simulink model "WTPG"  (R2022a)
settings: Solver=FixedStepDiscrete  StartTime=0.0  StopTime=10  FixedStep=0.04  RelTol=1e-3  EnableMultiTasking=on
PreLoadFcn:
  | listing = dir;
  | if (contains([listing .name], 'TCAF')) && (contains([listing .name], 'MAP'))
  |     addpath('./TCAF', './MAP');
  |     addpath( genpath('./MAP') );
  | elseif (contains([listing .name], 'WTPG.slx'))
  |     addpath('../TCAF', '../MAP');
  |     addpath( genpath('../MAP') );
  | else
  | 
  | end
  | 
  | load('BusStructureWTPG.mat');
  | load('TRN\BusStructureTRN.mat');
InitFcn:
  | listing = dir;
  | if (contains([listing .name], 'TCAF')) && (contains([listing .name], 'MAP'))
  |     addpath('./TCAF', './MAP');
  |     addpath( genpath('./MAP') );
  | elseif (contains([listing .name], 'WTPG.slx'))
  |     addpath('../TCAF', '../MAP');
  |     addpath( genpath('../MAP') );
  | else
  | 
  | end
  | 
  | load('BusStructureWTPG.mat');
  | load('TRN\BusStructureTRN.mat');
values from neighbouring files (symbols this model uses):
  isFeasible = logsout{idx_WTPGDatapump}.Values.isFeasible.Data(ii,:)    [WTPG_SIM_AFTERPLOT.m]
  wtpgOffTerMap = logsout{idx_WTPGOutput}.Values.wtpgOffTerMap.Data(ii,:)    [WTPG_SIM_AFTERPLOT.m]
  wtpgValid = logsout{idx_WTPGOutput}.Values.wtpgValid.Data(ii)    [WTPG_SIM_AFTERPLOT.m]
undefined symbols (not defined in the file or in its folder): predictedTrajectory, wtp, wtpgOffObsMap, wtpValid
libraries: simulink x1
settings Model: Creator=ASCL  LastModifiedBy=ASCL
settings SolverCC: AutoInsertRateTranBlk=on
settings DataIOCC: SaveOutput=off  SignalLogging=off  DSMLogging=off  SaveTime=off  ReturnWorkspaceOutputs=off
settings OptimizationCC: BlockReduction=off  DefaultParameterBehavior=Inlined  UseDivisionForNetSlopeComputation=on  GainParamInheritBuiltInType=on  UseFloatMulNetSlope=on  ExpressionFolding=off  PassReuseOutputArgsAs=Individual arguments  ZeroExternalMemoryAtStartup=off  ZeroInternalMemoryAtStartup=off  EfficientFloat2IntCast=on  LifeSpan=inf  OptimizeBlockOrder=speed  DifferentSizesBufferReuse=on  EfficientTunableParamExpr=on
settings DebuggingCC: SignalInfNanChecking=warning  ReadBeforeWriteMsg=EnableAllAsError  WriteAfterWriteMsg=EnableAllAsError  WriteAfterReadMsg=EnableAllAsError  IntegerOverflowMsg=error  ParameterTunabilityLossMsg=error  UniqueDataStoreMsg=error  AssertControl=DisableAll  NonBusSignalsTreatedAsBus=error  SFInvalidInputDataAccessInChartInitDiag=error  SFTransitionOutsideNaturalParentDiag=error  SFUnreachableExecutionPathDiag=error  SFUndirectedBroadcastEventsDiag=error  IntegerSaturationMsg=error
settings HardwareCC: ProdBitPerPointer=32  ProdBitPerSizeT=32  ProdBitPerPtrDiffT=32  ProdLargestAtomicInteger=Long  ProdLargestAtomicFloat=Double  ProdEndianess=BigEndian  ProdWordSize=32  ProdLongLongMode=on  ProdHWDeviceType=Freescale->MPC83xx
settings ModelReferenceCC: ModelReferenceNumInstancesAllowed=Single
settings SFSimCC: SimCustomHeaderCode="#include \"MAP.h\""  SimUserSources=MAP.c  SimUserLibraries=WS2_32.LIB  CompileTimeRecursionLimit=0  EnableRuntimeRecursion=off  MATLABDynamicMemAlloc=off
settings RTWCC: SystemTargetFile=ert.tlc  TemplateMakefile=ert_default_tmf  GenerateReport=on  RTWUseSimCustomCode=on  CustomHeaderCode="#include \"MAP.h\""  CustomSource=MAP.c  CustomLibrary=WS2_32.LIB  BuildConfiguration=Faster Runs  IncludeHyperlinkInReport=on  LaunchReport=on  GenerateTraceInfo=on  GenerateTraceReport=on  GenerateTraceReportSl=on  GenerateTraceReportSf=on  GenerateTraceReportEml=on  GenerateCodeMetricsReport=on
settings CodeAppCC: ForceParamTrailComments=on  IgnoreCustomStorageClasses=off  OperatorAnnotations=on  SimulinkDataObjDesc=on  SFDataObjDesc=on  MATLABFcnDesc=on  InsertBlockDesc=on  StateflowObjectComments=on  MATLABSourceComments=on  EnableCustomComments=on  InlinedPrmAccess=Macros  ReqsInCode=on
settings ERTTargetCC: TargetLangStandard=C99 (ISO)  UtilityFuncGeneration=Shared location  GenerateSampleERTMain=on  IncludeMdlTerminateFcn=off  CombineSignalStateStructs=on  SuppressErrorStatus=on  SupportAbsoluteTime=off  SupportNonFinite=off  SupportComplex=off  SupportVariableSizeSignals=on  ParenthesesLevel=Standards  CastingMode=Standards  GenerateSharedConstants=off  InlinedParameterPlacement=NonHierarchical  ERTCustomFileTemplate=example_file_process.tlc  RateTransitionBlockCode=Function  PreserveIfCondition=on  ConvertIfToSwitch=off  EnableSignedLeftShifts=off  EnableSignedRightShifts=off

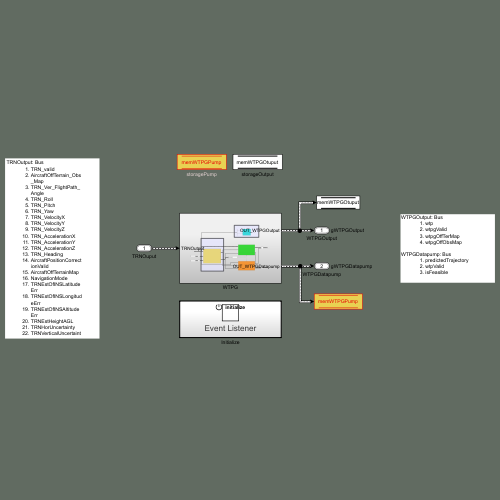
[thumbnail: Simulink's stored preview of the top-level diagram]
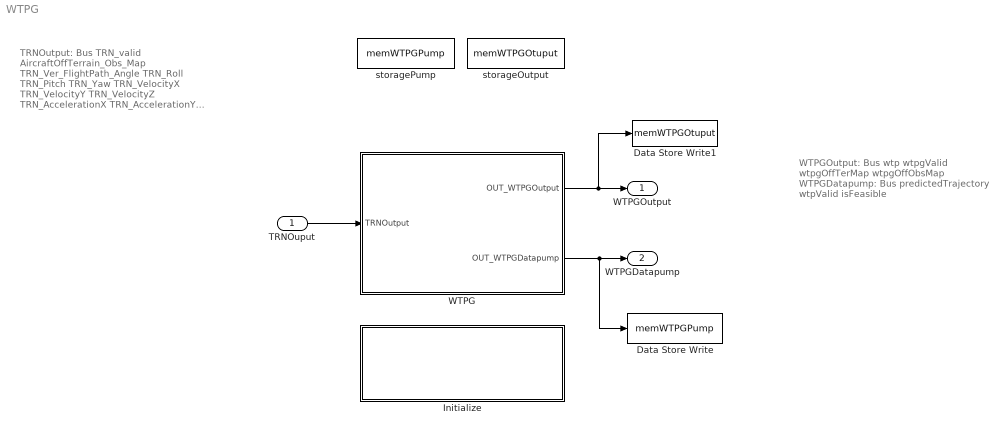
== system WTPG ==
  note: TRNOutput: Bus
      | TRN_valid
      | AircraftOffTerrain_Obs_Map
      | TRN_Ver_FlightPath_Angle
      | TRN_Roll
      | TRN_Pitch
      | TRN_Yaw
      | TRN_VelocityX
      | TRN_VelocityY
      | TRN_VelocityZ
      | TRN_AccelerationX
      | TRN_AccelerationY
      | TRN_AccelerationZ
      | TRN_Heading
      | AircraftPositionCorrectionValid
      | AircraftOffTerrainMap
      | NavigationMode
      | TRNEstOfINSLatitudeErr
      | TRNEstOfINSLongitudeErr
      | TRNEstOfINSAltitudeErr
      | TRNEstHeightAGL
      | TRNHorUncertainty
      | TRNVerticalUncertainty
      | TRNTimeTag
      | Latitude_INS
      | Longitude_INS
      | Altitude_INS
  note: WTPGOutput: Bus
      | wtp
      | wtpgValid
      | wtpgOffTerMap
      | wtpgOffObsMap
      |
      | WTPGDatapump: Bus
      | predictedTrajectory
      | wtpValid
      | isFeasible
  TRNOuput : Inport  OutDataTypeStr=Bus: TRNOutput  SampleTime=0.04  Interpolate=off  BusOutputAsStruct=on
  Data Store Write : DataStoreWrite  DataStoreName=memWTPGPump  IndexOptions=Index vector (dialog)  Indices=1  OutputSizes=1
  Data Store Write1 : DataStoreWrite  DataStoreName=memWTPGOtuput  IndexOptions=Index vector (dialog)  Indices=1  OutputSizes=1
  Initialize : Subsystem  TreatAsAtomicUnit=on
  WTPG : Subsystem
  storageOutput : DataStoreMemory  DataStoreName=memWTPGOtuput  WriteAfterWriteMsg=warning  VectorParams1D=off  ShowAdditionalParam=off  OutDataTypeStr=Bus: WTPGOutput
      settings: LockScale=on
  storagePump : DataStoreMemory  DataStoreName=memWTPGPump  WriteAfterWriteMsg=warning  VectorParams1D=off  ShowAdditionalParam=off  OutDataTypeStr=Bus: WTPGDatapump
      settings: LockScale=on
  WTPGOutput : Outport  SignalName=gWTPGOutput  OutDataTypeStr=Bus: WTPGOutput  SampleTime=0.04  BusOutputAsStruct=on
  WTPGDatapump : Outport  Port=2  SignalName=gWTPGDatapump  OutDataTypeStr=Bus: WTPGDatapump  SampleTime=0.04  BusOutputAsStruct=on
  wires:
  TRNOuput/1 -> WTPG/1(TRNOutput)
  WTPG/1(OUT_WTPGOutput) -> Data Store Write1/1, WTPGOutput/1
  WTPG/2(OUT_WTPGDatapump) -> Data Store Write/1, WTPGDatapump/1

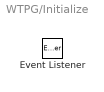
== system WTPG/Initialize ==
  Event Listener : EventListener  DisableCoverage=on  EventName=reset

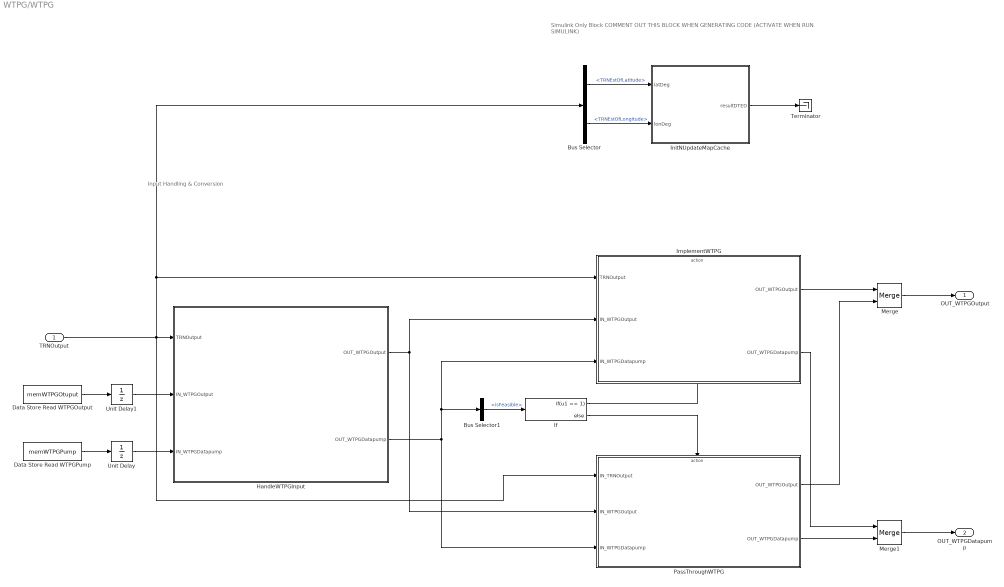
== system WTPG/WTPG ==
  note: Simulink Only Block
      | COMMENT OUT THIS BLOCK WHEN GENERATING CODE
      | (ACTIVATE WHEN RUN SIMULINK)
  note: Input Handling & Conversion
  TRNOutput : Inport  OutDataTypeStr=Bus: TRNOutput
  Bus Selector : BusSelector  OutputSignals=TRNEstOfLatitude,TRNEstOfLongitude
  Bus Selector1 : BusSelector  OutputSignals=isFeasible
  Data Store Read WTPGPump : DataStoreRead  DataStoreName=memWTPGPump  IndexOptions=Index vector (dialog)  Indices=1  OutputSizes=1
  Data Store Read WTPGOutput : DataStoreRead  DataStoreName=memWTPGOtuput  IndexOptions=Index vector (dialog)  Indices=1  OutputSizes=1
  HandleWTPGInput : Subsystem  TreatAsAtomicUnit=on
      settings: RTWSystemCode=Nonreusable function  RTWFcnNameOpts=Use subsystem name  FunctionInterfaceSpec=Allow arguments (Optimized)
  If : If  IfExpression=u1 == 1
  ImplementWTPG : Subsystem
      settings: RTWSystemCode=Nonreusable function  RTWFcnNameOpts=Use subsystem name
  InitNUpdateMapCache : Subsystem  TreatAsAtomicUnit=on
  Merge : Merge
  Merge1 : Merge
  PassThroughWTPG : Subsystem  TreatAsAtomicUnit=on
      settings: RTWSystemCode=Nonreusable function  RTWFcnNameOpts=Use subsystem name
  Terminator : Terminator
  Unit Delay : UnitDelay  SampleTime=-1  HasFrameUpgradeWarning=on
  Unit Delay1 : UnitDelay  SampleTime=-1  HasFrameUpgradeWarning=on
  OUT_WTPGOutput : Outport  OutDataTypeStr=Bus: WTPGOutput  SampleTime=0.04
  OUT_WTPGDatapump : Outport  Port=2  OutDataTypeStr=Bus: WTPGDatapump  SampleTime=0.04
  wires:
  InitNUpdateMapCache/1(resultDTED) -> Terminator/1
  ImplementWTPG/1(OUT_WTPGOutput) -> Merge/1
  ImplementWTPG/2(OUT_WTPGDatapump) -> Merge1/1
  Bus Selector/1 -> InitNUpdateMapCache/1(latDeg)  "<TRNEstOfLatitude>"
  Bus Selector/2 -> InitNUpdateMapCache/2(lonDeg)  "<TRNEstOfLongitude>"
  Data Store Read WTPGOutput/1 -> Unit Delay1/1
  Data Store Read WTPGPump/1 -> Unit Delay/1
  Unit Delay1/1 -> HandleWTPGInput/2(IN_WTPGOutput)
  Unit Delay/1 -> HandleWTPGInput/3(IN_WTPGDatapump)
  HandleWTPGInput/2(OUT_WTPGDatapump) -> ImplementWTPG/3(IN_WTPGDatapump), Bus Selector1/1, PassThroughWTPG/3(IN_WTPGDatapump)
  HandleWTPGInput/1(OUT_WTPGOutput) -> ImplementWTPG/2(IN_WTPGOutput), PassThroughWTPG/2(IN_WTPGOutput)
  Bus Selector1/1 -> If/1  "<isFeasible>"
  If/2 -> PassThroughWTPG/Action
  If/1 -> ImplementWTPG/Action
  TRNOutput/1 -> PassThroughWTPG/1(IN_TRNOutput), Bus Selector/1, ImplementWTPG/1(TRNOutput), HandleWTPGInput/1(TRNOutput)
  PassThroughWTPG/1(OUT_WTPGOutput) -> Merge/2
  Merge/1 -> OUT_WTPGOutput/1
  PassThroughWTPG/2(OUT_WTPGDatapump) -> Merge1/2
  Merge1/1 -> OUT_WTPGDatapump/1

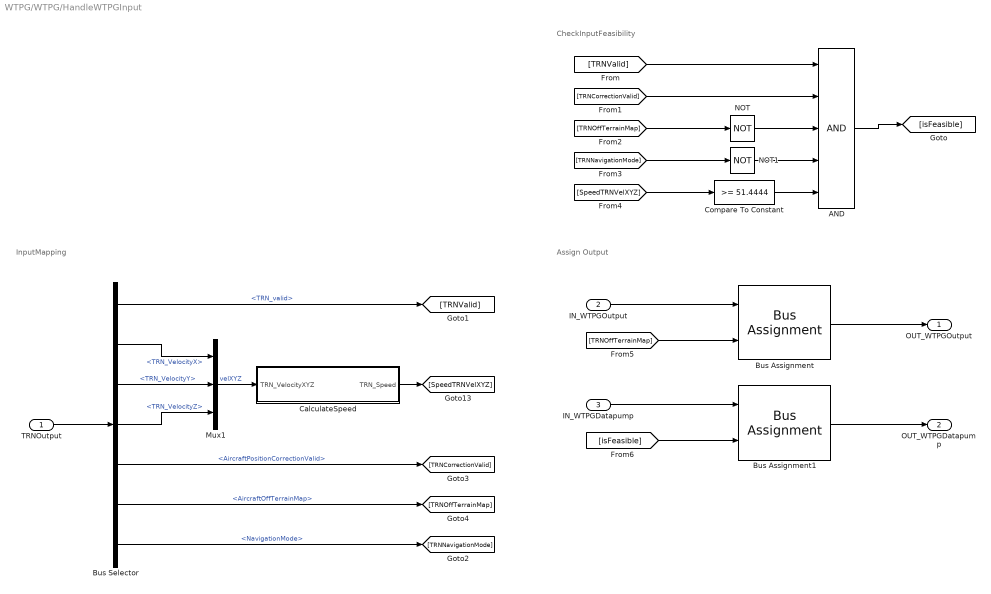
== system WTPG/WTPG/HandleWTPGInput ==
  note: Assign Output
  note: CheckInputFeasibility
  note: InputMapping
  TRNOutput : Inport  OutDataTypeStr=Bus: TRNOutput  SampleTime=0.04
  IN_WTPGOutput : Inport  Port=2
  IN_WTPGDatapump : Inport  Port=3
  AND : Logic  Inputs=5  AllPortsSameDT=off  OutDataTypeStr=boolean
  Bus Assignment : BusAssignment  AssignedSignals=wtpgOffTerMap
  Bus Assignment1 : BusAssignment  AssignedSignals=isFeasible
  Bus Selector : BusSelector  OutputSignals=TRN_valid,TRN_VelocityX,TRN_VelocityY,TRN_VelocityZ,AircraftPositionCorrectionValid,AircraftOffTerrainMap,NavigationMode
  CalculateSpeed : Subsystem
  Compare To Constant : simulink/Logic and Bit Operations/Compare To Constant  relop=>=  const=51.4444  OutDataTypeStr=boolean
  Mux1 : Mux  Inputs=3
  NOT : Logic  Operator=NOT  AllPortsSameDT=off  OutDataTypeStr=boolean
  NOT1 : Logic  Operator=NOT  AllPortsSameDT=off  OutDataTypeStr=boolean
  OUT_WTPGOutput : Outport
  OUT_WTPGDatapump : Outport  Port=2
  wires:
  TRNOutput/1 -> Bus Selector/1
  Bus Selector/2 -> Mux1/1  "<TRN_VelocityX>"
  Mux1/1 -> CalculateSpeed/1(TRN_VelocityXYZ)  "velXYZ"
  Bus Selector/4 -> Mux1/3  "<TRN_VelocityZ>"
  Bus Selector/3 -> Mux1/2  "<TRN_VelocityY>"
  Bus Selector/1 -> [TRNValid]  "<TRN_valid>"
  Bus Selector/5 -> [TRNCorrectionValid]  "<AircraftPositionCorrectionValid>"
  Bus Selector/6 -> [TRNOffTerrainMap]  "<AircraftOffTerrainMap>"
  Bus Selector/7 -> [TRNNavigationMode]  "<NavigationMode>"
  [TRNOffTerrainMap] -> NOT/1
  [TRNValid] -> AND/1
  [TRNCorrectionValid] -> AND/2
  NOT/1 -> AND/3
  [TRNNavigationMode] -> NOT1/1
  AND/1 -> [isFeasible]
  NOT1/1 -> AND/4
  CalculateSpeed/1(TRN_Speed) -> [SpeedTRNVelXYZ]
  [SpeedTRNVelXYZ] -> Compare To Constant/1
  Compare To Constant/1 -> AND/5
  IN_WTPGOutput/1 -> Bus Assignment/1
  Bus Assignment/1 -> OUT_WTPGOutput/1
  [TRNOffTerrainMap] -> Bus Assignment/2
  IN_WTPGDatapump/1 -> Bus Assignment1/1
  Bus Assignment1/1 -> OUT_WTPGDatapump/1
  [isFeasible] -> Bus Assignment1/2

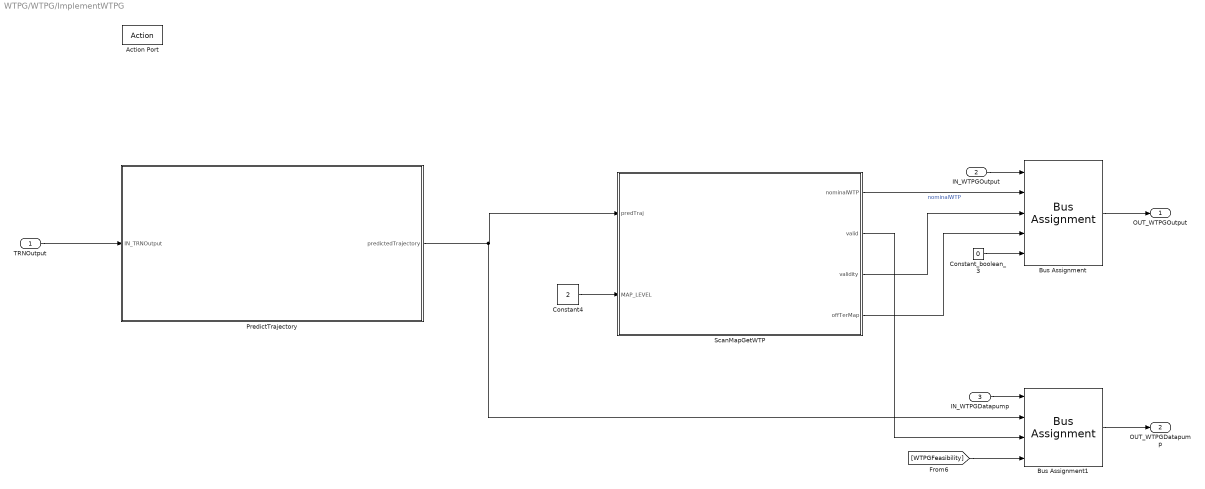
== system WTPG/WTPG/ImplementWTPG ==
  TRNOutput : Inport
  IN_WTPGOutput : Inport  Port=2  OutDataTypeStr=Bus: WTPGOutput
  IN_WTPGDatapump : Inport  Port=3  OutDataTypeStr=Bus: WTPGDatapump
  Action Port : ActionPort  ActionPortLabel=if(u1 == 1)
  Bus Assignment : BusAssignment  AssignedSignals=wtp,wtpgValid,wtpgOffTerMap,wtpgOffObsMap
  Bus Assignment1 : BusAssignment  AssignedSignals=predictedTrajectory,wtpValid,isFeasible
  Constant4 : Constant  Value=2  OutDataTypeStr=uint16  SampleTime=0.04
  Constant_boolean_3 : Constant  Value=0  OutDataTypeStr=boolean  SampleTime=0.04
  PredictTrajectory : Subsystem
  ScanMapGetWTP : MATLAB Function  TreatAsAtomicUnit=on  SystemSampleTime=0.04
      settings: RTWSystemCode=Nonreusable function  RTWFcnNameOpts=Use subsystem name
  OUT_WTPGOutput : Outport  OutDataTypeStr=Bus: WTPGOutput
  OUT_WTPGDatapump : Outport  Port=2  OutDataTypeStr=Bus: WTPGDatapump  SampleTime=0.04
  wires:
  ScanMapGetWTP/3(validity) -> Bus Assignment/3
  PredictTrajectory/1(predictedTrajectory) -> Bus Assignment1/2, ScanMapGetWTP/1(predTraj)
  Constant4/1 -> ScanMapGetWTP/2(MAP_LEVEL)
  Bus Assignment/1 -> OUT_WTPGOutput/1
  ScanMapGetWTP/1(nominalWTP) -> Bus Assignment/2  "nominalWTP"
  Constant_boolean_3/1 -> Bus Assignment/5
  ScanMapGetWTP/4(offTerMap) -> Bus Assignment/4
  IN_WTPGOutput/1 -> Bus Assignment/1
  IN_WTPGDatapump/1 -> Bus Assignment1/1
  [WTPGFeasibility] -> Bus Assignment1/4
  Bus Assignment1/1 -> OUT_WTPGDatapump/1
  ScanMapGetWTP/2(valid) -> Bus Assignment1/3
  TRNOutput/1 -> PredictTrajectory/1(IN_TRNOutput)

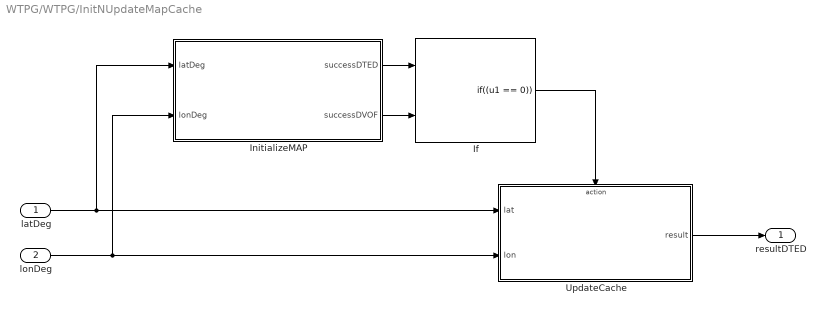
== system WTPG/WTPG/InitNUpdateMapCache ==
  latDeg : Inport  OutDataTypeStr=double
  lonDeg : Inport  Port=2  OutDataTypeStr=double
  If : If  NumInputs=2  IfExpression=(u1 == 0)  ShowElse=off
  InitializeMAP : MATLAB Function  TreatAsAtomicUnit=on
  UpdateCache : Subsystem  TreatAsAtomicUnit=on
  resultDTED : Outport  VectorParamsAs1DForOutWhenUnconnected=off
  wires:
  lonDeg/1 -> InitializeMAP/2(lonDeg), UpdateCache/2(lon)
  UpdateCache/1(result) -> resultDTED/1
  InitializeMAP/1(successDTED) -> If/1
  latDeg/1 -> InitializeMAP/1(latDeg), UpdateCache/1(lat)
  InitializeMAP/2(successDVOF) -> If/2
  If/1 -> UpdateCache/Action

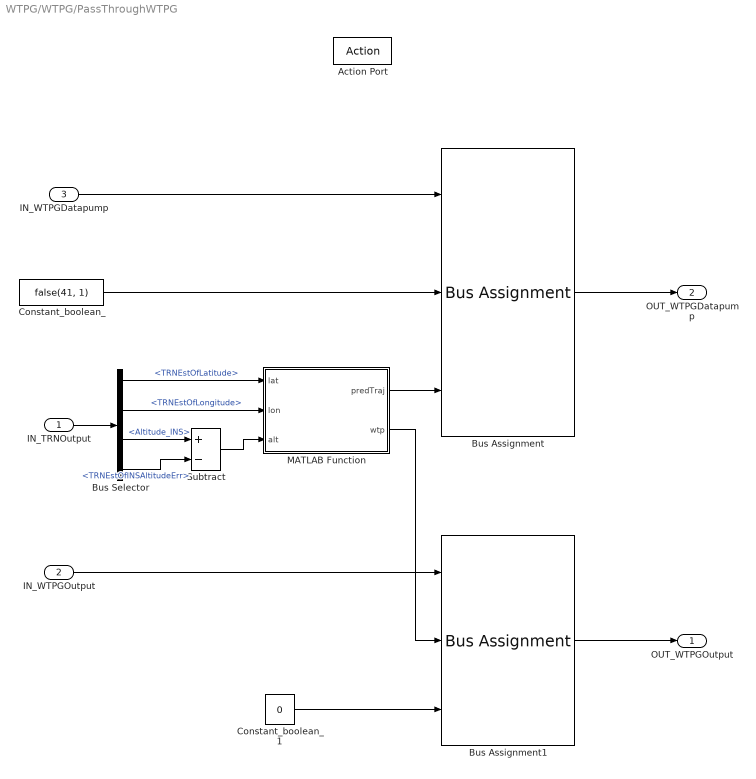
== system WTPG/WTPG/PassThroughWTPG ==
  IN_TRNOutput : Inport  OutDataTypeStr=Bus: TRNOutput
  IN_WTPGOutput : Inport  Port=2  OutDataTypeStr=Bus: WTPGOutput
  IN_WTPGDatapump : Inport  Port=3  OutDataTypeStr=Bus: WTPGDatapump
  Action Port : ActionPort  ActionPortLabel=else
  Bus Assignment : BusAssignment  AssignedSignals=wtpValid,predictedTrajectory
  Bus Assignment1 : BusAssignment  AssignedSignals=wtp,wtpgValid
  Bus Selector : BusSelector  OutputSignals=TRNEstOfLatitude,TRNEstOfLongitude,Altitude_INS,TRNEstOfINSAltitudeErr
  Constant_boolean_ : Constant  Value=false(41, 1)  OutDataTypeStr=boolean
  Constant_boolean_1 : Constant  Value=0  OutDataTypeStr=boolean
  MATLAB Function : MATLAB Function  TreatAsAtomicUnit=on
  Subtract : Sum  Inputs=+-
  OUT_WTPGOutput : Outport  OutDataTypeStr=Bus: WTPGOutput
  OUT_WTPGDatapump : Outport  Port=2  OutDataTypeStr=Bus: WTPGDatapump
  wires:
  IN_WTPGDatapump/1 -> Bus Assignment/1
  Bus Assignment/1 -> OUT_WTPGDatapump/1
  Constant_boolean_/1 -> Bus Assignment/2
  MATLAB Function/1(predTraj) -> Bus Assignment/3
  IN_TRNOutput/1 -> Bus Selector/1
  Bus Selector/2 -> MATLAB Function/2(lon)  "<TRNEstOfLongitude>"
  Bus Selector/1 -> MATLAB Function/1(lat)  "<TRNEstOfLatitude>"
  Bus Selector/3 -> Subtract/1  "<Altitude_INS>"
  Bus Selector/4 -> Subtract/2  "<TRNEstOfINSAltitudeErr>"
  Subtract/1 -> MATLAB Function/3(alt)
  IN_WTPGOutput/1 -> Bus Assignment1/1
  Bus Assignment1/1 -> OUT_WTPGOutput/1
  MATLAB Function/2(wtp) -> Bus Assignment1/2
  Constant_boolean_1/1 -> Bus Assignment1/3

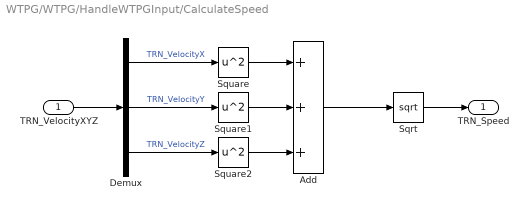
== system WTPG/WTPG/HandleWTPGInput/CalculateSpeed ==
  TRN_VelocityXYZ : Inport
  Add : Sum  Inputs=+++
  Demux : Demux  Outputs=3
  Sqrt : Sqrt
  Square : Math  Operator=square  SignedPower=on  RndMeth=Zero
  Square1 : Math  Operator=square  SignedPower=on  RndMeth=Zero
  Square2 : Math  Operator=square  SignedPower=on  RndMeth=Zero
  TRN_Speed : Outport
  wires:
  Demux/1 -> Square/1  "TRN_VelocityX"
  Demux/3 -> Square2/1  "TRN_VelocityZ"
  Demux/2 -> Square1/1  "TRN_VelocityY"
  Square/1 -> Add/1
  Square1/1 -> Add/2
  Square2/1 -> Add/3
  Add/1 -> Sqrt/1
  Sqrt/1 -> TRN_Speed/1
  TRN_VelocityXYZ/1 -> Demux/1

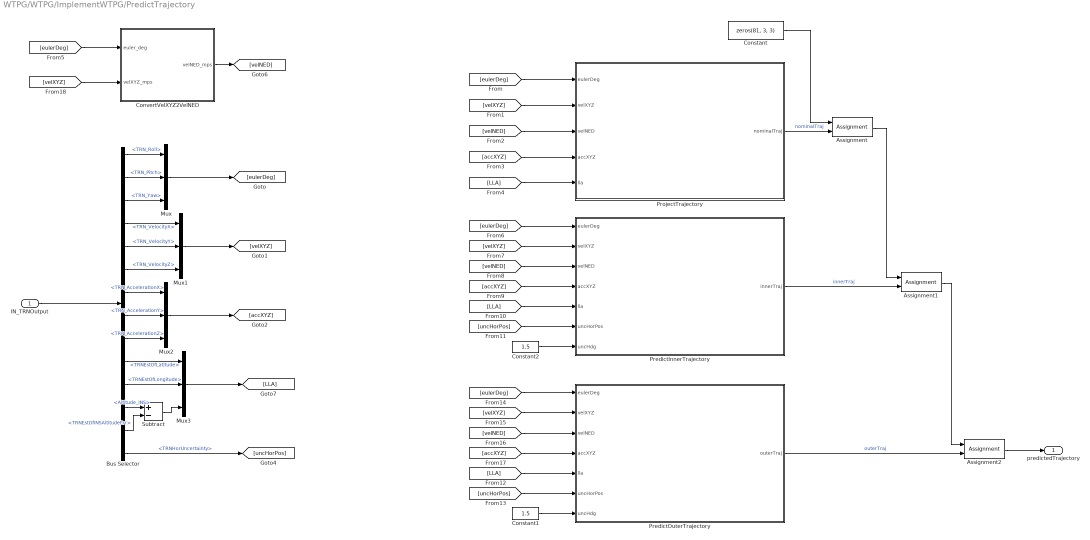
== system WTPG/WTPG/ImplementWTPG/PredictTrajectory ==
  IN_TRNOutput : Inport  OutDataTypeStr=Bus: TRNOutput
  Assignment : Assignment  NumberOfDimensions=3  DiagnosticForDimensions=Warning  IndexOptions=Assign all,Index vector (dialog),Assign all  Indices=1,1,1  OutputSizes=1,1,1
  Assignment1 : Assignment  NumberOfDimensions=3  DiagnosticForDimensions=Warning  IndexOptions=Assign all,Index vector (dialog),Assign all  Indices=1,2,1  OutputSizes=1,1,1
  Assignment2 : Assignment  NumberOfDimensions=3  DiagnosticForDimensions=Warning  IndexOptions=Assign all,Index vector (dialog),Assign all  Indices=1,3,1  OutputSizes=1,1,1
  Bus Selector : BusSelector  OutputSignals=TRN_Roll,TRN_Pitch,TRN_Yaw,TRN_VelocityX,TRN_VelocityY,TRN_VelocityZ,TRN_AccelerationX,TRN_AccelerationY,TRN_AccelerationZ,TRNEstOfLatitude,TRNEstOfLongitude,Altitude_INS,TRNEstOfINSAltitudeErr,TRNHorUncertainty
  Constant : Constant  Value=zeros(81, 3, 3)  OutDataTypeStr=double  SampleTime=0.04
  Constant1 : Constant  Value=1.5  SampleTime=0.04
  Constant2 : Constant  Value=1.5  SampleTime=0.04
  ConvertVelXYZ2VelNED : MATLAB Function  TreatAsAtomicUnit=on  SystemSampleTime=0.04
  Mux{,1..3} (4 alike) : Mux  Inputs=3
  PredictInnerTrajectory : MATLAB Function  TreatAsAtomicUnit=on  SystemSampleTime=0.04
      settings: RTWSystemCode=Nonreusable function  RTWFcnNameOpts=Use subsystem name  FunctionInterfaceSpec=Allow arguments (Match graphical interface)
  PredictOuterTrajectory : MATLAB Function  TreatAsAtomicUnit=on  SystemSampleTime=0.04
      settings: RTWSystemCode=Nonreusable function  RTWFcnNameOpts=Use subsystem name  FunctionInterfaceSpec=Allow arguments (Match graphical interface)
  ProjectTrajectory : MATLAB Function  TreatAsAtomicUnit=on  SystemSampleTime=0.04
      settings: RTWSystemCode=Nonreusable function  RTWFcnNameOpts=Use subsystem name  FunctionInterfaceSpec=Allow arguments (Match graphical interface)
  Subtract : Sum  Inputs=+-
  predictedTrajectory : Outport  SampleTime=0.04
  wires:
  Constant/1 -> Assignment/1
  ProjectTrajectory/1(nominalTraj) -> Assignment/2  "nominalTraj"
  Assignment/1 -> Assignment1/1
  PredictInnerTrajectory/1(innerTraj) -> Assignment1/2  "innerTraj"
  Assignment1/1 -> Assignment2/1
  PredictOuterTrajectory/1(outerTraj) -> Assignment2/2  "outerTraj"
  Assignment2/1 -> predictedTrajectory/1
  [uncHorPos] -> PredictOuterTrajectory/6(uncHorPos)
  [LLA] -> PredictOuterTrajectory/5(lla)
  [accXYZ] -> PredictOuterTrajectory/4(accXYZ)
  [velNED] -> PredictOuterTrajectory/3(velNED)
  [velXYZ] -> PredictOuterTrajectory/2(velXYZ)
  [eulerDeg] -> PredictOuterTrajectory/1(eulerDeg)
  [eulerDeg] -> ProjectTrajectory/1(eulerDeg)
  [velXYZ] -> ProjectTrajectory/2(velXYZ)
  [velNED] -> ProjectTrajectory/3(velNED)
  [accXYZ] -> ProjectTrajectory/4(accXYZ)
  [LLA] -> ProjectTrajectory/5(lla)
  Constant2/1 -> PredictInnerTrajectory/7(uncHdg)
  [uncHorPos] -> PredictInnerTrajectory/6(uncHorPos)
  [LLA] -> PredictInnerTrajectory/5(lla)
  [accXYZ] -> PredictInnerTrajectory/4(accXYZ)
  [velNED] -> PredictInnerTrajectory/3(velNED)
  [velXYZ] -> PredictInnerTrajectory/2(velXYZ)
  [eulerDeg] -> PredictInnerTrajectory/1(eulerDeg)
  Constant1/1 -> PredictOuterTrajectory/7(uncHdg)
  IN_TRNOutput/1 -> Bus Selector/1
  Bus Selector/1 -> Mux/1  "<TRN_Roll>"
  Bus Selector/2 -> Mux/2  "<TRN_Pitch>"
  Bus Selector/3 -> Mux/3  "<TRN_Yaw>"
  Mux/1 -> [eulerDeg]
  Bus Selector/5 -> Mux1/2  "<TRN_VelocityY>"
  Bus Selector/4 -> Mux1/1  "<TRN_VelocityX>"
  Bus Selector/6 -> Mux1/3  "<TRN_VelocityZ>"
  Mux1/1 -> [velXYZ]
  ConvertVelXYZ2VelNED/1(velNED_mps) -> [velNED]
  [eulerDeg] -> ConvertVelXYZ2VelNED/1(euler_deg)
  [velXYZ] -> ConvertVelXYZ2VelNED/2(velXYZ_mps)
  Bus Selector/7 -> Mux2/1  "<TRN_AccelerationX>"
  Bus Selector/8 -> Mux2/2  "<TRN_AccelerationY>"
  Bus Selector/9 -> Mux2/3  "<TRN_AccelerationZ>"
  Mux2/1 -> [accXYZ]
  Mux3/1 -> [LLA]
  Bus Selector/10 -> Mux3/1  "<TRNEstOfLatitude>"
  Bus Selector/11 -> Mux3/2  "<TRNEstOfLongitude>"
  Bus Selector/12 -> Subtract/1  "<Altitude_INS>"
  Bus Selector/13 -> Subtract/2  "<TRNEstOfINSAltitudeErr>"
  Subtract/1 -> Mux3/3
  Bus Selector/14 -> [uncHorPos]  "<TRNHorUncertainty>"

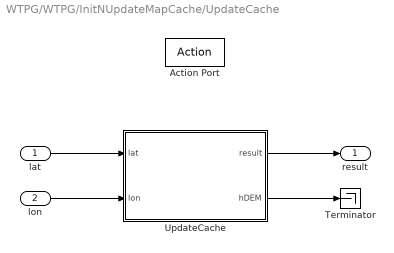
== system WTPG/WTPG/InitNUpdateMapCache/UpdateCache ==
  lat : Inport
  lon : Inport  Port=2
  Action Port : ActionPort  ActionPortLabel=if((u1 == 0))
  Terminator : Terminator
  UpdateCache : MATLAB Function  TreatAsAtomicUnit=on
  result : Outport  VectorParamsAs1DForOutWhenUnconnected=off
  wires:
  UpdateCache/1(result) -> result/1
  lat/1 -> UpdateCache/1(lat)
  lon/1 -> UpdateCache/2(lon)
  UpdateCache/2(hDEM) -> Terminator/1

== matlab function WTPG/InitNUpdateMapCache/InitializeMAP ==
  data: successDTED output; successDVOF output; latDeg input; lonDeg input
function [successDTED, successDVOF] = InitializeMAP(latDeg, lonDeg)
%InitializeMAP

% Persistent variable
persistent firstRun
if isempty(firstRun)
    firstRun = true;
end

% Initialize output
flagDTED = int32(1);
flagDVOF = int32(1);
successDTED = int32(1);
successDVOF = int32(1);
hDEM = 0.0;

if firstRun
    % Path of DTED data
    pathDTED = 'C:\Users\ASCL\Documents\GitHub\DTNS\MAP\MAP_DB';

    % Length of DETD data path
    strLenDTED = int32(strlength(pathDTED));
    
    hDEM = coder.ceval('MAPGetTerrainHeight', latDeg, lonDeg);
    if IsNear(hDEM, -1.0)
        % Call [ InitialMap ] : 맵 폴더 위치 설정
        flagDTED = coder.ceval('InitialMap', pathDTED, strLenDTED );
        successDTED = flagDTED;
        if (~successDTED)
            firstRun = false;
        end
    else
        successDTED = int32(0);
        firstRun = false;       
    end
else
    successDTED = int32(0);
    successDVOF = int32(0);
end

== matlab function WTPG/ImplementWTPG/PredictTrajectory/ProjectTrajectory ==
  data: nominalTraj output; eulerDeg input; velXYZ input; velNED input; accXYZ input; lla input
function nominalTraj = ProjectTrajectory(eulerDeg, velXYZ, velNED, accXYZ, lla)
%ProjectTrajectory 예측 비행경로를 생성
% 예측 비행경로 배열을 생성 (81, 1, 3)

persistent DELTA_T

% Define constants
if isempty(DELTA_T)
    DELTA_T = 0.25;
end

% Define constants
GRAV_ACC = 9.8;
LIMIT_TAN_ROL = 4;
LIMIT_TURN_RATE = 0.222; % [rad/s]
RAD2DEG = 180/pi;
ALONG_TRACK_STEPS = 81;

% Initialize Predicted Trajectory
nominalTraj = zeros(ALONG_TRACK_STEPS, 1, 3);

% Input Handling
rol = eulerDeg(1);
pit = eulerDeg(2);
hdg = eulerDeg(3);

velX = velXYZ(1);
velY = velXYZ(2);
velZ = velXYZ(3);

velN = velNED(1);
velE = velNED(2);
velD = velNED(3);

lat = lla(1);
lon = lla(2);
alt = lla(3);

% Flight path angle (deg)
gamma = atan2d(-velD, sqrt(velN^2+velE^2));

% Inertial speed
iSpd = sqrt( velX^2 + velY^2 + velZ^2 );
    
% Saturate inertial speed (since TAS is unavailable, use inertial spd) 
iSpd = saturate(iSpd, 75.1089, 500);

% Calculate the length of a degree
[latLength, lonLength] = getLengthOfADegree(lat, alt);
velLat = velN / latLength;
velLon = velE / lonLength;

% Start point
nominalTraj(1, 1, 1) = lat;
nominalTraj(1, 1, 2) = lon;
nominalTraj(1, 1, 3) = alt;

for ii = 2:ALONG_TRACK_STEPS
    
    % [1] Update Attitude
    
    % Saturate tangent of roll (max bank angle = 75.9630 deg)
    tanRol = saturate(tand(rol), -LIMIT_TAN_ROL, LIMIT_TAN_ROL);

    % Saturate inertial speed (since TAS is unavailable, use inertial spd) 
    iSpd = saturate(iSpd, 75.1089, 500);
    
    % Calculate turn rate [rad/s]
    turnRate = GRAV_ACC * tanRol / iSpd;
    
    % Saturate turn rate 
    turnRate = saturate(turnRate, -LIMIT_TURN_RATE, LIMIT_TURN_RATE);
        
    % Update heading [deg]
    hdg = hdg + turnRate * DELTA_T * RAD2DEG;
    
    % Update Flight Path Angle [deg]
    %        reaction time: 1.5 sec
    %        rate of change: 10 deg/s
    if ii < 4
        gamma = gamma;
    elseif gamma < -(10*DELTA_T)
        gamma = gamma + 10 * DELTA_T;
    elseif gamma < 0.0
        gamma = 0.0;
    else
        gamma = gamma;
    end

    % [2] Update Velocity
    velNTmp = sqrt(velN^2+velE^2+velD^2)*cosd(hdg)*cosd(gamma);
    velE    = sqrt(velN^2+velE^2+velD^2)*sind(hdg)*cosd(gamma);
    velN    = velNTmp;
    velDOld = velD;
    velD    = - sqrt(velN^2+velE^2+velD^2)*sind(gamma);

    % [3] Update Position
    % Rate of change in geodetic coordinates [deg/s]
    [latLength, lonLength] = getLengthOfADegree(nominalTraj(ii, 1, 1), nominalTraj(ii, 1, 3));

    velLatOld = velLat;
    velLonOld = velLon;
    velLat  = velN / latLength;
    velLon  = velE / lonLength;
    
    nominalTraj(ii, 1, 1) = nominalTraj(ii-1, 1, 1) + (velLat + velLatOld)/2 * DELTA_T;
    nominalTraj(ii, 1, 2) = nominalTraj(ii-1, 1, 2) + (velLon + velLonOld)/2 * DELTA_T;
    nominalTraj(ii, 1, 3) = nominalTraj(ii-1, 1, 3) - (velD + velDOld)/2 * DELTA_T;

end

end

%% Internal Functions

function [latLength, lonLength] = getLengthOfADegree(lat, h)
%GETLENGTHOFADEGREE
% Calculate the length of one degree of both latitude and longitude
% for a specified latitude and height
%
% == Inputs =========
% lat               - Latitude [deg]
% h                 - Height [m]
% 
% == Outputs ========
% latLength         - Length of 1 deg of latitude on the ref. spheroid [m]
% lonLength         - Length of 1 deg of longitude on the ref. spheroid [m]
% ===================
%%%%%%%%%%%%%%%%%%%%%%%%%%%%%%%%%%%%%%%%%%%%%%%%%%%%%%%%%%%%%%%%%%%%%%%%%%%

% WGS84 Parameters
eRadius = 6378137.0;
eEccen = 0.08181919;

% Radius of curvature in prime vertical
nE = eRadius / sqrt( 1 - (eEccen^2*(sind(lat))^2) );
% Meridian Radius of Curavature
mE = eRadius * (1 - eEccen^2) / (1 - eEccen^2*(sind(lat))^2)^(1.5);

lonLength = (nE + h) * cosd(lat) * (pi/180);
latLength = (mE + h) * (pi/180);

end

function out = saturate(in, minVal, maxVal)
%SATURATE
% Saturates input value to [min, max]
%
% == Inputs =========
% in                - input value
% minVal            - minimum value
% maxVal            - maximum value
% == Outputs ========
% out               - saturated output value
% ===================

out = min(maxVal, max(minVal, in));

end

== matlab function WTPG/ImplementWTPG/PredictTrajectory/PredictInnerTrajectory ==
  data: innerTraj output; eulerDeg input; velXYZ input; velNED input; accXYZ input; lla input; uncHorPos input; uncHdg input
function innerTraj = PredictInnerTrajectory(eulerDeg, velXYZ, velNED, accXYZ, lla, uncHorPos, uncHdg)
%PredictInnerTrajectory 예측 비행경로를 생성
% 예측 비행경로 배열을 생성 (ALONG_TRACK_STEPS, 3, 3)
%       - Assumption 1: current aircraft state has uncertainty (3-sigma)
persistent DELTA_T
% Define constants
if isempty(DELTA_T)
    DELTA_T = 0.25;
end
GRAV_ACC = 9.8;
LIMIT_TAN_ROL = 4;
LIMIT_TURN_RATE = 0.222; % [rad/s]
RAD2DEG = 180/pi;
ALONG_TRACK_STEPS = 81;

% Constants for compare floating-point numbers
TOL = eps(0.5);

% Input Handling
rol = eulerDeg(1);
pit = eulerDeg(2);
hdg = eulerDeg(3);

velX = velXYZ(1);
velY = velXYZ(2);
velZ = velXYZ(3);

velN = velNED(1);
velE = velNED(2);
velD = velNED(3);

lat = lla(1);
lon = lla(2);
alt = lla(3);

% Flight path angle (deg)
gamma = atan2d(-velD, sqrt(velN^2+velE^2));

% Inertial speed
velXRef = sqrt( velX^2 + velY^2 + velZ^2 );

% Saturate inertial speed (since TAS is unavailable, use inertial spd)
velXRef = saturate(velXRef, 75.1089, 500);

% Saturate tangent of roll (max bank angle = 75.9630 deg)
tanRol = saturate(tand(rol), -LIMIT_TAN_ROL, LIMIT_TAN_ROL);

% Calculate turn rate [rad/s]
turnRate = GRAV_ACC * tanRol / velXRef;

% Saturate turn rate
turnRate = saturate(turnRate, -LIMIT_TURN_RATE, LIMIT_TURN_RATE);

% hdg = hdg + turnRate * RAD2DEG * 1;

% Saturate Uncertainties 
uncHorPos = saturate(uncHorPos, 35.56, 228.6);
uncHdg = saturate(uncHdg, 0.1, 5);

% Direction of uncertaitny addition
isTurnRight = (0 <= eulerDeg(1)) && (eulerDeg(1) < 180);
if isTurnRight
    uncPosRot = 90;
else
    uncHdg = (-1) * uncHdg;
    uncPosRot = -90;
end

% 3-sigma uncertainty for Heading
unitDirection = [velN; velE; 0] / norm([velN; velE; 0]);
unitDirection = rotateZ(3*uncHdg) * unitDirection;
hdg = hdg + 3*uncHdg;

% Update Velocity
velRef = sqrt(velN^2+velE^2+velD^2);
velN   = velRef*cosd(hdg)*cosd(gamma);
%         velNTmp = sqrt(velN^2+velE^2+velD^2)*cosd(hdg)*cosd(gamma);
velE    = velRef*sind(hdg)*cosd(gamma);
%         velN    = velNTmp;
velDOld = velD;
%         velD    = - sqrt(velN^2+velE^2+velD^2)*sind(gamma);
velD    = - velRef*sind(gamma);

% 3-sigma uncertainty for position
delPos = 3 * uncHorPos * rotateZ(uncPosRot + turnRate * RAD2DEG * 1) * unitDirection;

% Calculate the length of a degree
[latLength, lonLength] = getLengthOfADegree(lat, alt);
velLat  = velN / latLength;
velLon  = velE / lonLength;

% Initialize Predicted Trajectory
innerTraj = zeros(ALONG_TRACK_STEPS, 1, 3);

% Start point
innerTraj(1, 1, 1) = lat + delPos(1)/latLength;
innerTraj(1, 1, 2) = lon + delPos(2)/lonLength;
innerTraj(1, 1, 3) = alt;

for ii = 2:ALONG_TRACK_STEPS

    curT = (ii -1 ) * DELTA_T;

    if curT <= 20
        % [1] Update Attitude
        % Saturate tangent of roll (max bank angle = 75.9630 deg)
        tanRol = saturate(tand(rol), -LIMIT_TAN_ROL, LIMIT_TAN_ROL);

        % Saturate inertial speed (since TAS is unavailable, use inertial spd)
        velXRef = saturate(velXRef, 75.1089, 360.111);

        % Calculate turn rate [rad/s]
        turnRate = GRAV_ACC * tanRol / velXRef;

        % Saturate turn rate
        turnRate = saturate(turnRate, -LIMIT_TURN_RATE, LIMIT_TURN_RATE);

        % Update heading [deg]
        hdg = hdg + turnRate * DELTA_T * RAD2DEG;

        % Update Flight Path Angle [deg]
        %        reaction time: 1.5 sec
        %        rate of change: 10 deg/s
        if ii < 4
            gamma = gamma;
        elseif gamma < -(10*DELTA_T)
            gamma = gamma + 10 * DELTA_T;
        elseif gamma < 0.0
            gamma = 0.0;
        else
            gamma = gamma;
        end

        % [2] Update Velocity
        velRef = sqrt(velN^2+velE^2+velD^2);
        velN   = velRef*cosd(hdg)*cosd(gamma);
%         velNTmp = sqrt(velN^2+velE^2+velD^2)*cosd(hdg)*cosd(gamma);
        velE    = velRef*sind(hdg)*cosd(gamma);
%         velN    = velNTmp;
        velDOld = velD;
%         velD    = - sqrt(velN^2+velE^2+velD^2)*sind(gamma);
        velD    = - velRef*sind(gamma);
    else
        % [1] Update Attitude
        % No update

        % Update Flight Path Angle [deg]
        %        reaction time: 1.5 sec
        %        rate of change: 10 deg/s
        if ii < 4
            gamma = gamma;
        elseif gamma < -(10*DELTA_T)
            gamma = gamma + 10 * DELTA_T;
        elseif gamma < 0.0
            gamma = 0.0;
        else
            gamma = gamma;
        end

        % [2] Update Velocity
        velRef = sqrt(velN^2+velE^2+velD^2);
        velN   = velRef*cosd(hdg)*cosd(gamma);
%         velNTmp = sqrt(velN^2+velE^2+velD^2)*cosd(hdg)*cosd(gamma);
        velE    = velRef*sind(hdg)*cosd(gamma);
%         velN    = velNTmp;
        velDOld = velD;
%         velD    = - sqrt(velN^2+velE^2+velD^2)*sind(gamma);
        velD    = - velRef*sind(gamma);
    end

    % [3] Update Position
    % Rate of change in geodetic coordinates [deg/s]
    if abs( mod(ii, 41) - 0) < TOL % mod(ii, 41) == 0
        [latLength, lonLength] = getLengthOfADegree(innerTraj(ii, 1, 1), innerTraj(ii, 1, 3));
    end
    velLatOld = velLat;
    velLonOld = velLon;
    velLat  = velN / latLength;
    velLon  = velE / lonLength;

    innerTraj(ii, 1, 1) = innerTraj(ii-1, 1, 1) + (velLat + velLatOld)/2 * DELTA_T;
    innerTraj(ii, 1, 2) = innerTraj(ii-1, 1, 2) + (velLon + velLonOld)/2 * DELTA_T;
    innerTraj(ii, 1, 3) = innerTraj(ii-1, 1, 3) - (velD + velDOld)/2 * DELTA_T;

end

end

%% Internal Functions
function R = rotateZ(ang)
%ROTATEZ
% Rotation matrix for rotations around z-axis
% R = rotateZ(ang) creates a 3-by-3 matrix used to rotate a 3-by-1 vector
% or 3-by-N matrix of vectors around the z-axis by ang degrees.

%     R = zeros(3,3);
assert( isscalar(ang));
    
    R = [cosd(ang), -sind(ang), 0; ...
         sind(ang), cosd(ang),  0; ...
         0,         0,          1];
    
end

function [latLength, lonLength] = getLengthOfADegree(lat, h)
%GETLENGTHOFADEGREE
% Calculate the length of one degree of both latitude and longitude
% for a specified latitude and height
%
% == Inputs =========
% lat               - Latitude [deg]
% h                 - Height [m]
% 
% == Outputs ========
% latLength         - Length of 1 deg of latitude on the ref. spheroid [m]
% lonLength         - Length of 1 deg of longitude on the ref. spheroid [m]
% ===================
%%%%%%%%%%%%%%%%%%%%%%%%%%%%%%%%%%%%%%%%%%%%%%%%%%%%%%%%%%%%%%%%%%%%%%%%%%%

% WGS84 Parameters
eRadius = 6378137.0;
eEccen = 0.08181919;

% Radius of curvature in prime vertical
nE = eRadius / sqrt( 1 - (eEccen^2*(sind(lat))^2) );
% Meridian Radius of Curavature
mE = eRadius * (1 - eEccen^2) / (1 - eEccen^2*(sind(lat))^2)^(1.5);

lonLength = (nE + h) * cosd(lat) * (pi/180);
latLength = (mE + h) * (pi/180);

end

function out = saturate(in, minVal, maxVal)
%SATURATE
% Saturates input value to [min, max]
%
% == Inputs =========
% in                - input value
% minVal            - minimum value
% maxVal            - maximum value
% == Outputs ========
% out               - saturated output value
% ===================

out = min(maxVal, max(minVal, in));

end

== matlab function WTPG/ImplementWTPG/PredictTrajectory/PredictOuterTrajectory ==
  data: outerTraj output; eulerDeg input; velXYZ input; velNED input; accXYZ input; lla input; uncHorPos input; uncHdg input
function outerTraj = PredictOuterTrajectory(eulerDeg, velXYZ, velNED, accXYZ, lla, uncHorPos, uncHdg)
%PredictOuterTrajectory 예측 비행경로를 생성

persistent DELTA_T

% Define constants
if isempty(DELTA_T)
    DELTA_T = 0.25;
end
GRAV_ACC = 9.8;
ALONG_TRACK_STEPS = 81;

% Input Handling
rol = eulerDeg(1);
pit = eulerDeg(2);
hdg = eulerDeg(3);

velX = velXYZ(1);
velY = velXYZ(2);
velZ = velXYZ(3);

velN = velNED(1);
velE = velNED(2);
velD = velNED(3);

lat = lla(1);
lon = lla(2);
alt = lla(3);

% Flight path angle (deg)
gamma = atan2d(-velD, sqrt(velN^2+velE^2));

% Saturate Uncertainties 
uncHorPos = saturate(uncHorPos, 35.56, 228.6);
uncHdg = saturate(uncHdg, 0.1, 5);

% Direction of uncertaitny addition
isTurnRight = (0 <= eulerDeg(1)) && (eulerDeg(1) < 180);
if isTurnRight
    uncHdg = (-1) * uncHdg;
    uncPosRot = -90;
else
    uncPosRot = 90;
end

% 3-sigma uncertainty for Heading
unitDirection = [velN; velE; 0] / norm([velN; velE; 0]);
unitDirection = rotateZ(3*uncHdg) * unitDirection;
hdg = hdg + 3*uncHdg;

% Update Velocity
velRef = sqrt(velN^2+velE^2+velD^2);
velN   = velRef*cosd(hdg)*cosd(gamma);
%         velNTmp = sqrt(velN^2+velE^2+velD^2)*cosd(hdg)*cosd(gamma);
velE    = velRef*sind(hdg)*cosd(gamma);
%         velN    = velNTmp;
velDOld = velD;
%         velD    = - sqrt(velN^2+velE^2+velD^2)*sind(gamma);
velD    = - velRef*sind(gamma);

% 3-sigma uncertainty for position
delPos = 3 * uncHorPos * rotateZ(uncPosRot) * unitDirection;

% Calculate the length of a degree
[latLength, lonLength] = getLengthOfADegree(lat, alt);
velLat  = velN / latLength;
velLon  = velE / lonLength;

% Initialize Predicted Trajectory
outerTraj = zeros(ALONG_TRACK_STEPS, 1, 3);

% Start point
outerTraj(1, 1, 1) = lat + delPos(1)/latLength;
outerTraj(1, 1, 2) = lon + delPos(2)/lonLength;
outerTraj(1, 1, 3) = alt;

rolRate = 120;
keepT = 2.5;

stage = [ floor(keepT/DELTA_T) + 1, ...
          floor(keepT/DELTA_T) + 1 + floor( (abs(rol)/rolRate)/DELTA_T ) + 1];

velXRef = saturate(velX, 75.1089, 360.111);

for ii = 2:ALONG_TRACK_STEPS
    
    if (stage(1) < ii) && (ii <= stage(2))
        % [2] roll recovery
        
        % Update Attitude
        % (roll)
        rol_old = rol;
        if abs(rol-0) <= abs(rolRate*DELTA_T)
            rol_new = 0;
        else
            rol_new = sign(rol) * (abs(rol) - rolRate*DELTA_T);
        end
        
        % (heading)
        if ( abs( tand(rol_old) ) > 4 )
            hdg = hdg + ...
                0.5 * ( GRAV_ACC * 4 * sign( tand(rol_old) ) / velXRef * DELTA_T) * 180/pi +...
                0.5 * ( GRAV_ACC * 4 * sign( tand(rol_new) ) / velXRef * DELTA_T) * 180/pi; 
        else
            hdg = hdg + ...
                0.5 * ( GRAV_ACC * tand(rol_old) / velXRef * DELTA_T) * 180/pi + ...
                0.5 * ( GRAV_ACC * tand(rol_new) / velXRef * DELTA_T) * 180/pi;
        end
        rol = rol_new;

        % Update Flight Path Angle [deg]
        %        reaction time: 1.5 sec
        %        rate of change: 10 deg/s
        if ii < 4
            gamma = gamma;
        elseif gamma < -(10*DELTA_T)
            gamma = gamma + 10 * DELTA_T;
        elseif gamma < 0.0
            gamma = 0.0;
        else
            gamma = gamma;
        end
        
        % [2] Update Velocity
        velRef = sqrt(velN^2+velE^2+velD^2);
        velN   = velRef*cosd(hdg)*cosd(gamma);
        %         velNTmp = sqrt(velN^2+velE^2+velD^2)*cosd(hdg)*cosd(gamma);
        velE    = velRef*sind(hdg)*cosd(gamma);
        %         velN    = velNTmp;
        velDOld = velD;
        %         velD    = - sqrt(velN^2+velE^2+velD^2)*sind(gamma);
        velD    = - velRef*sind(gamma);
        
        % Rate of change in geodetic coordinates [deg/s]
        [latLength, lonLength] = getLengthOfADegree(outerTraj(ii, 1, 1), outerTraj(ii, 1, 3));
        velLatOld = velLat;
        velLonOld = velLon;
        velLat  = velN / latLength;
        velLon  = velE / lonLength;
    
        outerTraj(ii, 1, 1) = outerTraj(ii-1, 1, 1) + (velLat + velLatOld)/2 * DELTA_T;
        outerTraj(ii, 1, 2) = outerTraj(ii-1, 1, 2) + (velLon + velLonOld)/2 * DELTA_T;
        outerTraj(ii, 1, 3) = outerTraj(ii-1, 1, 3) - (velD + velDOld)/2 * DELTA_T;
        
    else
        % [1] in Pilot reaction time
        % [3] wing-level flight

        % Update Attitude
        if ( abs( tand(rol) ) > 4 ) && ( abs(velX) > 0.1 )
            hdg = hdg + ( GRAV_ACC * 4 * sign( tand(rol) ) / velX * DELTA_T) * 180/pi; 
        elseif ( abs( tand(rol) ) <= 4 ) && ( abs(velX) > 0.1 )
            hdg = hdg + ( GRAV_ACC * tand(rol) / velX * DELTA_T) * 180/pi;
        else
            hdg = hdg + ( GRAV_ACC * tand(rol) / 0.1 * DELTA_T) * 180/pi;
        end
        
        % Update Flight Path Angle [deg]
        %        reaction time: 1.5 sec
        %        rate of change: 10 deg/s
        if ii < 4
            gamma = gamma;
        elseif gamma < -(10*DELTA_T)
            gamma = gamma + 10 * DELTA_T;
        elseif gamma < 0.0
            gamma = 0.0;
        else
            gamma = gamma;
        end
        
        % [2] Update Velocity
        velRef = sqrt(velN^2+velE^2+velD^2);
        velN   = velRef*cosd(hdg)*cosd(gamma);
        %         velNTmp = sqrt(velN^2+velE^2+velD^2)*cosd(hdg)*cosd(gamma);
        velE    = velRef*sind(hdg)*cosd(gamma);
        %         velN    = velNTmp;
        velDOld = velD;
        %         velD    = - sqrt(velN^2+velE^2+velD^2)*sind(gamma);
        velD    = - velRef*sind(gamma);
        % Rate of change in geodetic coordinates [deg/s]
        [latLength, lonLength] = getLengthOfADegree(outerTraj(ii, 1, 1), outerTraj(ii, 1, 3));

        velLatOld = velLat;
        velLonOld = velLon;
        velLat  = velN / latLength;
        velLon  = velE / lonLength;

        outerTraj(ii, 1, 1) = outerTraj(ii-1, 1, 1) + (velLat + velLatOld)/2 * DELTA_T;
        outerTraj(ii, 1, 2) = outerTraj(ii-1, 1, 2) + (velLon + velLonOld)/2 * DELTA_T;
        outerTraj(ii, 1, 3) = outerTraj(ii-1, 1, 3) - (velD + velDOld)/2 * DELTA_T;

    end

end


end

%% Internal Functions
function R = rotateZ(ang)
%ROTATEZ
% Rotation matrix for rotations around z-axis
% R = rotateZ(ang) creates a 3-by-3 matrix used to rotate a 3-by-1 vector
% or 3-by-N matrix of vectors around the z-axis by ang degrees.

%     R = zeros(3,3);
assert( isscalar(ang));
    
    R = [cosd(ang), -sind(ang), 0; ...
         sind(ang), cosd(ang),  0; ...
         0,         0,          1];
    
end

function [latLength, lonLength] = getLengthOfADegree(lat, h)
%GETLENGTHOFADEGREE
% Calculate the length of one degree of both latitude and longitude
% for a specified latitude and height
%
% == Inputs =========
% lat               - Latitude [deg]
% h                 - Height [m]
% 
% == Outputs ========
% latLength         - Length of 1 deg of latitude on the ref. spheroid [m]
% lonLength         - Length of 1 deg of longitude on the ref. spheroid [m]
% ===================
%%%%%%%%%%%%%%%%%%%%%%%%%%%%%%%%%%%%%%%%%%%%%%%%%%%%%%%%%%%%%%%%%%%%%%%%%%%

% WGS84 Parameters
eRadius = 6378137.0;
eEccen = 0.08181919;

% Radius of curvature in prime vertical
nE = eRadius / sqrt( 1 - (eEccen^2*(sind(lat))^2) );
% Meridian Radius of Curavature
mE = eRadius * (1 - eEccen^2) / (1 - eEccen^2*(sind(lat))^2)^(1.5);

lonLength = (nE + h) * cosd(lat) * (pi/180);
latLength = (mE + h) * (pi/180);

end

function out = saturate(in, minVal, maxVal)
%SATURATE
% Saturates input value to [min, max]
%
% == Inputs =========
% in                - input value
% minVal            - minimum value
% maxVal            - maximum value
% == Outputs ========
% out               - saturated output value
% ===================

out = min(maxVal, max(minVal, in));

end

== matlab function WTPG/ImplementWTPG/PredictTrajectory/ConvertVelXYZ2VelNED ==
  data: euler_deg input; velNED_mps output; velXYZ_mps input
function velNED_mps = ConvertVelXYZ2VelNED(euler_deg, velXYZ_mps)
%ConvertVelXYZ2VelNED

% Initialize
velNED_mps  = zeros(3,1);

% Define constants
r2d = 180/pi;

% Body to NED
cRol = cosd(euler_deg(1));
sRol = sind(euler_deg(1));
cPit = cosd(euler_deg(2));
sPit = sind(euler_deg(2));
cYaw = cosd(euler_deg(3));
sYaw = sind(euler_deg(3));

% Coordinate Transformation
C_b_n   = [ cPit*cYaw, sRol*sPit*cYaw-cRol*sYaw, cRol*sPit*cYaw+sRol*sYaw;...
            cPit*sYaw, sRol*sPit*sYaw+cRol*cYaw, cRol*sPit*sYaw-sRol*cYaw;...
                -sPit,                sRol*cPit,                cRol*cPit];
% NED Velocity
velNED_mps = C_b_n * velXYZ_mps;

== matlab function WTPG/ImplementWTPG/ScanMapGetWTP ==
  data: nominalWTP output; valid output; predTraj input; validity output; offTerMap output; MAP_LEVEL input
function [nominalWTP, valid, validity, offTerMap] = ScanMapGetWTP(predTraj, MAP_LEVEL)
%ScanMapGetWTP 지형지물 탐색 및 WTP 생성
% 입력받은 예측 비행경로를 이용해 지형지물 정보를 탐색하고 WCP를 생성한다
%
%   [nominalWTP, valid] = ScanMapGetWTP(predTraj)
%
% INPUT
% - predTraj(ALONG_TRACK_STEPS, 3, 3)
%  *ALONG_TRACK_STEPS = 81
% - MAP_LEVEL
%
% OUTPUT
% - nominalWTP(41, 1) : WTP array (0:0.5:20)
% - valid(41, 1)
% - validity
% - offTerMap

% DEFINE CONSTANTS
% RESOLUTION = double(1.0);
RESOLUTION = double(3.0);
% if (MAP_LEVEL == uint16(1))
%     RESOLUTION = double(3.0);
% elseif (MAP_LEVEL == uint16(2))
%     RESOLUTION = double(1.0);
% else
%     RESOLUTION = double(3.0);
% end
ARCSEC2DEG = 0.000277777777777777;
RESDEG = RESOLUTION * ARCSEC2DEG;

% Initialize
nominalWTP = zeros(41, 1, 'single');
valid = zeros(41, 1, 'logical');
validity = false;
offTerMap = false;

dist = 0.0;
dx = 0.0;
dy = 0.0;


% For every 0.5 sec (from 0 to 20 sec)
for ii = 1:2:size(predTraj, 1)

    % Initialize current & highest elevation
    highestElev = 0.0;
    curElev = 0.0;

    % Configure High and Low Indices
    if ii == 1
        lo = ii;
        hi = ii+1;
    elseif ii == size(predTraj, 1)
        lo = ii-1;
        hi = ii;
    else
        lo = ii-1;
        hi = ii+1;
    end

    % Position of Trapezoid. [Lat, Lon, Height]
    trapezoid = ...
        [ predTraj(lo, 2, 1), predTraj(lo, 2, 2) ...
        ; predTraj(hi, 2, 1), predTraj(hi, 2, 2) ...
        ; predTraj(hi, 3, 1), predTraj(hi, 3, 2) ...
        ; predTraj(lo, 3, 1), predTraj(lo, 3, 2) ...
        ; predTraj(lo, 2, 1), predTraj(lo, 2, 2)];
    
    % Bounding box coordinated at map post
    bBox = [min(trapezoid); max(trapezoid)];
    bBox = [...
        floor(bBox(1,:)/RESDEG)*RESDEG; ...
        ceil( bBox(2,:)/RESDEG)*RESDEG];

    % number of map post
    bBoxLatNum = round(abs((bBox(2,1)-bBox(1,1)) / RESDEG));
    bBoxLonNum = round(abs((bBox(2,2)-bBox(1,2)) / RESDEG));

    for jj = 0:bBoxLatNum
        for kk = 0:bBoxLonNum

            lat = bBox(1,1) + (bBox(2,1)-bBox(1,1))/bBoxLatNum * (jj);
            lon = bBox(1,2) + (bBox(2,2)-bBox(1,2))/bBoxLonNum * (kk);

            isIn = inpolygon(lat, lon, trapezoid(:,1), trapezoid(:,2));

            if ~isIn
                [dist, dx, dy] = distFromPoly(lat, lon, trapezoid(:,1), trapezoid(:,2));

                isAround = ...
                    ( dist - RESDEG < 0) ...
                    | ( (dx - RESDEG < 0) & (dy - RESDEG <0) );

                if isAround
                else
                    continue
                end
            else
            end

            curElev = coder.ceval('MAPGetTerrainHeight', lat, lon);
            if curElev == -1.0
                offTerMap = true;
            elseif curElev > highestElev
                highestElev = curElev;
            else
            end
        end
    end

    % Update
    nominalWTP((ii-1)/2+1, 1) = single(highestElev);
    valid((ii-1)/2+1, 1) = ~offTerMap;

end

validity = all(valid(1:11, 1));

end
% Internal functions
function [dist, dx, dy] = distFromPoly(x, y, xv, yv)
%distFromPoly
% INPUT
% -  x      : point's x coordinate
% -  y      : point's y coordinate
% -  xv     : vector of polygon vertices x coordinates
% -  yv     : vector of polygon vertices y coordinates
% * (xv, yv) should be closed!
%
% OUTPUT
% - dist    : distance from point to polygon (defined as a minimal distance from 
%       point to any of polygon's ribs, positive if the point is outside the
%       polygon and negative otherwise)
% - dx      : 
% - dy      : 
% -------------------------------------------------------------------------

dist = 0.0;
dx = 0.0;
dy = 0.0;
I = 0;
I2 = 0;
I3 = 0;

% linear parameters of segments that connect the vertices
% Ax + By + C = 0
A = -diff(yv);
B =  diff(xv);
C = yv(2:end).*xv(1:end-1) - xv(2:end).*yv(1:end-1);

% find the projection of point (x,y) on each rib
AB = 1./(A.^2 + B.^2);
vv = (A*x+B*y+C);
xp = x - (A.*AB).*vv;
yp = y - (B.*AB).*vv;

% Test for the case where a polygon rib is either horizontal or vertical
id_xv = find(diff(xv)==0);
xp(id_xv)=xv(id_xv);
id_yv = find(diff(yv)==0);
yp(id_yv)=yv(id_yv);

% find all cases where projected point is inside the segment
idx_x = (((xp>=xv(1:end-1)) & (xp<=xv(2:end))) | ((xp>=xv(2:end)) & (xp<=xv(1:end-1))));
idx_y = (((yp>=yv(1:end-1)) & (yp<=yv(2:end))) | ((yp>=yv(2:end)) & (yp<=yv(1:end-1))));
idx = idx_x & idx_y;

% distance from point (x,y) to the vertices
dv = sqrt((xv(1:end-1)-x).^2 + (yv(1:end-1)-y).^2);
if(~any(idx)) % all projections are outside of polygon ribs
    [dist,I] = min(dv);
    dx = abs(xv(I)-x);
    dy = abs(yv(I)-y);
else
    % distance from point (x,y) to the projection on ribs
    dp = sqrt((xp(idx)-x).^2 + (yp(idx)-y).^2);
    [min_dv,I] = min(dv);
    [min_dp,I2] = min(dp);
    [dist,I3] = min([min_dv min_dp]);
    if I3 == 1
        dx = abs(xv(I)-x);
        dy = abs(yv(I)-y);
    else
        dx = abs(xp(I2)-x);
        dy = abs(yp(I2)-y);
    end
end

if(inpolygon(x, y, xv, yv))
    dist = -dist;
end

end

== matlab function WTPG/PassThroughWTPG/MATLAB Function ==
  data: lat input; predTraj output; lon input; alt input; wtp output
function [predTraj, wtp] = createDummy(lat, lon, alt)

predTraj = zeros(81, 3, 3);
wtp = ones(41,1, 'single') * alt;

for ii = 1:size(predTraj, 1)
    for jj = 1:size(predTraj, 2)
        predTraj(ii, jj, 1) = lat;
        predTraj(ii, jj, 2) = lon;
        predTraj(ii, jj, 3) = alt;
    end
end

== matlab function WTPG/InitNUpdateMapCache/UpdateCache/UpdateCache ==
  data: result output; lat input; lon input; hDEM output
function [result, hDEM] = UpdateCache(lat, lon)
%UpdateCache

% Persistent variables
persistent latPrev lonPrev
if isempty(latPrev)
    latPrev = 0.0;
end
if isempty(lonPrev)
    lonPrev = 0.0;
end

hDEM = 0.0;

% Initialize output
result = int32(1);

if ( abs(lat - latPrev) > 0.05 ) || ( abs(lon - lonPrev) > 0.05)
    result = coder.ceval('UpdateCache', lat, lon);
    hDEM = coder.ceval('MAPGetTerrainHeight', lat, lon);

    if result == 0
        latPrev = lat;
        lonPrev = lon;
    end
else
    
end
